simulink model "error_ss"  (R2020b)
settings: Solver=VariableStepAuto  StartTime=0.0  StopTime=10  RelTol=1e-3
libraries: simulink x1
settings Model: Creator=cmparedes  LastModifiedBy=Acer

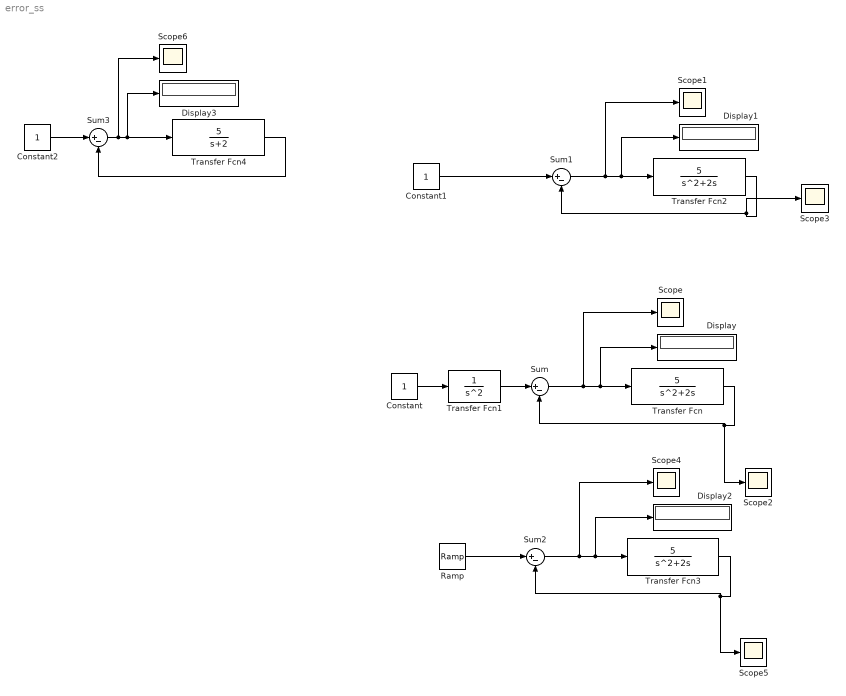
== system error_ss ==
  Constant : Constant
  Constant1 : Constant
  Constant2 : Constant
  Display{,1..3} (4 alike) : Display
  Ramp : simulink/Sources/Ramp  slope=6  start=0  InitialOutput=0
  Scope{,1..6} (7 alike) : Scope
  Sum{,1..3} (4 alike) : Sum  Inputs=|+-
  Transfer Fcn : TransferFcn  Numerator=[5]  Denominator=[1 2 0]
  Transfer Fcn1 : TransferFcn  Denominator=[1 0 0]
  Transfer Fcn2 : TransferFcn  Numerator=[5]  Denominator=[1 2 0]
  Transfer Fcn3 : TransferFcn  Numerator=[5]  Denominator=[1 2 0]
  Transfer Fcn4 : TransferFcn  Numerator=[5]  Denominator=[1 2]
  wires:
  Transfer Fcn/1 -> Sum/2, Scope2/1
  Sum/1 -> Scope/1, Display/1, Transfer Fcn/1
  Constant/1 -> Transfer Fcn1/1
  Transfer Fcn1/1 -> Sum/1
  Constant1/1 -> Sum1/1
  Sum1/1 -> Scope1/1, Display1/1, Transfer Fcn2/1
  Transfer Fcn2/1 -> Sum1/2, Scope3/1
  Ramp/1 -> Sum2/1
  Sum2/1 -> Scope4/1, Display2/1, Transfer Fcn3/1
  Transfer Fcn3/1 -> Sum2/2, Scope5/1
  Constant2/1 -> Sum3/1
  Sum3/1 -> Scope6/1, Display3/1, Transfer Fcn4/1
  Transfer Fcn4/1 -> Sum3/2
